simulink model "Robot4"  (R2018a)
settings: Solver=VariableStepAuto  StartTime=0.0  StopTime=10.0  RelTol=1e-3
settings Model: Creator=Carapinha  LastModifiedBy=Carapinha

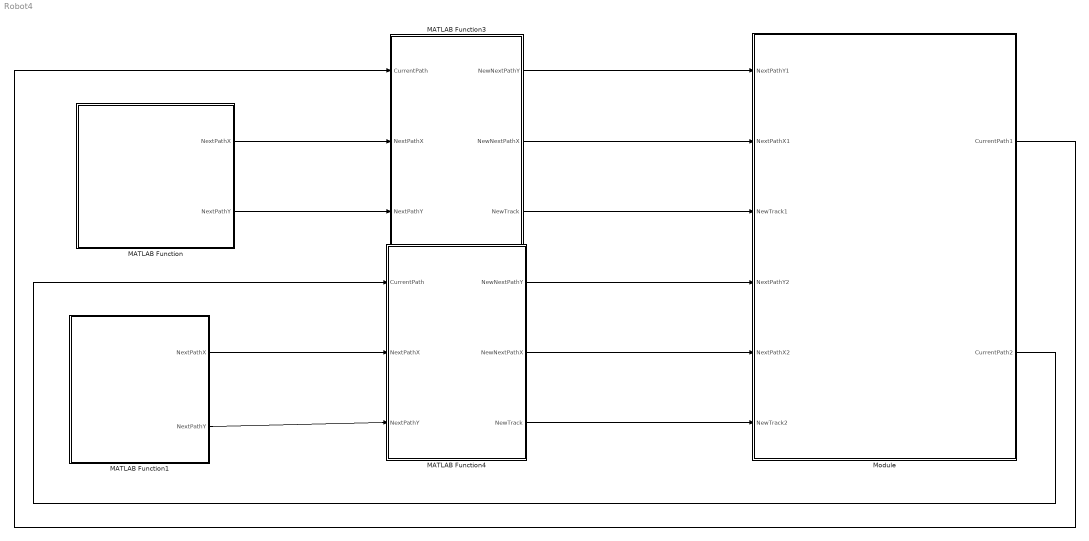
== system Robot4 ==
  MATLAB Function : MATLAB Function  TreatAsAtomicUnit=on
  MATLAB Function1 : MATLAB Function  TreatAsAtomicUnit=on
  MATLAB Function3 : MATLAB Function  TreatAsAtomicUnit=on
  MATLAB Function4 : MATLAB Function  TreatAsAtomicUnit=on
  Module : Stateflow chart  TreatAsAtomicUnit=on
  wires:
  MATLAB Function4/2(NewNextPathX) -> Module/5(NextPathX2)
  MATLAB Function4/1(NewNextPathY) -> Module/4(NextPathY2)
  MATLAB Function3/3(NewTrack) -> Module/3(NewTrack1)
  MATLAB Function1/2(NextPathY) -> MATLAB Function4/3(NextPathY)
  MATLAB Function3/1(NewNextPathY) -> Module/1(NextPathY1)
  MATLAB Function3/2(NewNextPathX) -> Module/2(NextPathX1)
  MATLAB Function1/1(NextPathX) -> MATLAB Function4/2(NextPathX)
  MATLAB Function/2(NextPathY) -> MATLAB Function3/3(NextPathY)
  Module/1(CurrentPath1) -> MATLAB Function3/1(CurrentPath)
  Module/2(CurrentPath2) -> MATLAB Function4/1(CurrentPath)
  MATLAB Function/1(NextPathX) -> MATLAB Function3/2(NextPathX)
  MATLAB Function4/3(NewTrack) -> Module/6(NewTrack2)

== matlab function Robot4/MATLAB Function1 ==
  data: NextPathX output; NextPathY output
function [NextPathX, NextPathY] = RandomPath()
    NextPathX = round(rand(1)*2-1);
    NextPathY = round(rand(1)*2-1);
    return
end

== matlab function Robot4/MATLAB Function ==
  data: NextPathX output; NextPathY output
function [NextPathX, NextPathY] = RandomPath()
    NextPathX = round(rand(1)*2-1);
    NextPathY = round(rand(1)*2-1);
    return
end

== stateflow chart Robot4/Module ==
  state Main
    state Robot1 [parallel]
      settings: executionOrder=1
      state StopR1
        entry:
        %PathBlocked
        Move1 = 1;
        Stop1 = 0;
      state MoveR1
        entry:
        Car1 = 1;
        Move1 = 0;
        Stop1 = 1;
      StopR1 -> MoveR1 [order 1] : [NewTrack1 == CurrentTrack2]
      (default) -> MoveR1
      MoveR1 -> StopR1 : [NewTrack1 ~= CurrentTrack2]
      StopR1 -> StopR1 [order 2] : [after(1,sec)]
    state Controller1 [parallel]
      settings: executionOrder=2
      state E
        entry:
        A(5,1) = 1;
        CurrentPath1 = 5;
        exit:
        A(5,1) = 0;
      state I
        entry:
        A(4,2) = 1;
        CurrentPath1 = 9;
        exit:
        A(4,2) = 0;
      state O
        entry:
        A(5,3) = 1;
        CurrentPath1 = 15;
        exit:
        A(5,3) = 0;
      state C
        entry:
        A(3,1) = 1;
        CurrentPath1 = 3;
        exit:
        A(3,1) = 0;
      state Start1
        entry:
      state S
        entry:
        A(4,4) = 1;
        CurrentPath1 = 19;
        exit:
        A(4,4) = 0;
      state A
        entry:
        A(1,1) = 1;
        CurrentPath1 = 1;
        exit:
        A(1,1) = 0;
      state G
        entry:
        A(2,2) = 1;
        CurrentPath1 = 7;
        exit:
        A(2,2) = 0;
      state M
        entry:
        A(3,3) = 1;
        CurrentPath1 = 13;
        exit:
        A(3,3) = 0;
      state Z
        entry:
        A(5,5) = 1;
        CurrentPath1 = 25;
        exit:
        A(5,5) = 0;
      state K
        entry:
        A(1,3) = 1;
        CurrentPath1 = 11;
        exit:
        A(1,3) = 0;
      state Q
        entry:
        A(2,4) = 1;
        CurrentPath1 = 17;
        exit:
        A(2,4) = 0;
      state X
        entry:
        A(3,5) = 1;
        CurrentPath1 = 23;
        exit:
        A(3,5) = 0;
      state U
        entry:
        A(1,5) = 1;
        CurrentPath1 = 21;
        exit:
        A(1,5) = 0;
      E -> Main.Controller1.I : [Move1 == 1 && NextPathX1 == -1 && NextPathY1 == -1]
      Main.Controller1.I -> E [order 2] : [Move1 == 1 && NextPathX1 == 1 && NextPathY1 == 1]
      (default) -> Start1
      Main.Controller1.C -> Main.Controller1.I [order 2] : [Move1 == 1 && NextPathX1 == 1 && NextPathY1 == -1]
      Main.Controller1.I -> Main.Controller1.O [order 3] : [Move1 == 1 && NextPathX1 == 1 && NextPathY1 == -1]
      Main.Controller1.I -> Main.Controller1.C [order 1] : [Move1 == 1 && NextPathX1 == -1 && NextPathY1 == 1]
      Main.Controller1.O -> Main.Controller1.I [order 1] : [Move1 == 1 && NextPathX1 == -1 && NextPathY1 == 1]
      Main.Controller1.C -> Main.Controller1.G [order 1] : [Move1 == 1 && NextPathX1 == -1 && NextPathY1 == -1]
      Main.Controller1.G -> Main.Controller1.C [order 2] : [Move1 == 1 && NextPathX1 == 1 && NextPathY1 == 1]
      Main.Controller1.O -> Main.Controller1.S [order 2] : [Move1 == 1 && NextPathX1 == -1 && NextPathY1 == -1]
      Main.Controller1.S -> Main.Controller1.O [order 2] : [Move1 == 1 && NextPathX1 == 1 && NextPathY1 == 1]
      Main.Controller1.I -> Main.Controller1.M [order 4] : [Move1 == 1 && NextPathX1 == -1 && NextPathY1 == -1]
      Main.Controller1.M -> Main.Controller1.I [order 1] : [Move1 == 1 && NextPathX1 == 1 && NextPathY1 == 1]
      Start1 -> Main.Controller1.A : [Car1 == 1]
      Main.Controller1.G -> Main.Controller1.M [order 3] : [Move1 == 1 && NextPathX1 == 1 && NextPathY1 == -1]
      Main.Controller1.A -> Main.Controller1.G : [Move1 == 1 && NextPathX1 == 1 && NextPathY1 == -1]
      Main.Controller1.S -> Main.Controller1.Z [order 3] : [Move1 == 1 && NextPathX1 == -1 && NextPathY1 == -1]
      Main.Controller1.S -> Main.Controller1.M [order 4] : [Move1 == 1 && NextPathX1 == -1 && NextPathY1 == 1]
      Main.Controller1.G -> Main.Controller1.A [order 1] : [Move1 == 1 && NextPathX1 == -1 && NextPathY1 == 1]
      Main.Controller1.M -> Main.Controller1.G [order 4] : [Move1 == 1 && NextPathX1 == -1 && NextPathY1 == 1]
      Main.Controller1.Z -> Main.Controller1.S : [Move1 == 1 && NextPathX1 == -1 && NextPathY1 == 1]
      Main.Controller1.M -> Main.Controller1.S [order 2] : [Move1 == 1 && NextPathX1 == 1 && NextPathY1 == -1]
      Main.Controller1.G -> Main.Controller1.K [order 4] : [Move1 == 1 && NextPathX1 == -1 && NextPathY1 == -1]
      Main.Controller1.K -> Main.Controller1.G [order 1] : [Move1 == 1 && NextPathX1 == 1 && NextPathY1 == 1]
      Main.Controller1.S -> Main.Controller1.X [order 1] : [Move1 == 1 && NextPathX1 == -1 && NextPathY1 == -1]
      Main.Controller1.X -> Main.Controller1.S [order 2] : [Move1 == 1 && NextPathX1 == 1 && NextPathY1 == 1]
      Main.Controller1.M -> Main.Controller1.Q [order 3] : [Move1 == 1 && NextPathX1 == -1 && NextPathY1 == -1]
      Main.Controller1.Q -> Main.Controller1.M [order 1] : [Move1 == 1 && NextPathX1 == 1 && NextPathY1 == 1]
      Main.Controller1.K -> Main.Controller1.Q [order 2] : [Move1 == 1 && NextPathX1 == 1 && NextPathY1 == -1]
      Main.Controller1.X -> Main.Controller1.Q [order 1] : [Move1 == 1 && NextPathX1 == -1 && NextPathY1 == 1]
      Main.Controller1.Q -> Main.Controller1.K [order 3] : [Move1 == 1 && NextPathX1 == -1 && NextPathY1 == 1]
      Main.Controller1.Q -> Main.Controller1.X [order 2] : [Move1 == 1 && NextPathX1 == 1 && NextPathY1 == -1]
      Main.Controller1.Q -> Main.Controller1.U [order 4] : [Move1 == 1 && NextPathX1 == -1 && NextPathY1 == -1]
      Main.Controller1.U -> Main.Controller1.Q : [Move1 == 1 && NextPathX1 == 1 && NextPathY1 == 1]
    state Robot4 [parallel]
      settings: executionOrder=3
      state StopR2
        entry:
        %PathBlocked
        Move2 = 1;
        Stop2 = 0;
      state MoveR2
        entry:
        Car2 = 1;
        Move2 = 0;
        Stop2 = 1;
      StopR2 -> MoveR2 [order 1] : [NewTrack2 == CurrentTrack1]
      (default) -> MoveR2
      MoveR2 -> StopR2 : [NewTrack2 ~= CurrentTrack1]
      StopR2 -> StopR2 [order 2] : [after(1,sec)]
    state Controller1 [parallel]
      settings: executionOrder=4
      state E1
        entry:
        A(5,1) = 2;
        CurrentPath2 = 5;
        exit:
        A(5,1) = 0;
      state C
        entry:
        A(3,1) = 2;
        CurrentPath2 = 3;
        exit:
        A(3,1) = 0;
      state I
        entry:
        A(4,2) = 2;
        CurrentPath2 = 9;
        exit:
        A(4,2) = 0;
      state O
        entry:
        A(5,3) = 2;
        CurrentPath2 = 15;
        exit:
        A(5,3) = 0;
      state Start2
        entry:
      state A
        entry:
        A(1,1) = 2;
        CurrentPath2 = 1;
        exit:
        A(1,1) = 0;
      state G
        entry:
        A(2,2) = 2;
        CurrentPath2 = 7;
        exit:
        A(2,2) = 0;
      state S
        entry:
        A(4,4) = 2;
        CurrentPath2 = 19;
        exit:
        A(4,4) = 0;
      state M
        entry:
        A(3,3) = 2;
        CurrentPath2 = 13;
        exit:
        A(3,3) = 0;
      state Z
        entry:
        A(5,5) = 2;
        CurrentPath2 = 25;
        exit:
        A(5,5) = 0;
      state Q
        entry:
        A(2,4) = 2;
        CurrentPath2 = 17;
        exit:
        A(2,4) = 0;
      state X
        entry:
        A(3,5) = 2;
        CurrentPath2 = 23;
        exit:
        A(3,5) = 0;
      state K
        entry:
        A(1,3) = 2;
        CurrentPath2 = 11;
        exit:
        A(1,3) = 0;
      state U
        entry:
        A(1,5) = 2;
        CurrentPath2 = 21;
        exit:
        A(1,5) = 0;
      Main.Controller1.I -> E1 [order 2] : [Move2 == 1 && NextPathX2 == 1 && NextPathY2 == 1]
      E1 -> Main.Controller1.I : [Move2 == 1 && NextPathX2 == -1 && NextPathY2 == -1]
      Main.Controller1.C -> Main.Controller1.I [order 2] : [Move2 == 1 && NextPathX2 == 1 && NextPathY2 == -1]
      (default) -> Start2
      Main.Controller1.I -> Main.Controller1.C [order 1] : [Move2 == 1 && NextPathX2 == -1 && NextPathY2 == 1]
      Main.Controller1.I -> Main.Controller1.O [order 3] : [Move2 == 1 && NextPathX2 == 1 && NextPathY2 == -1]
      Main.Controller1.C -> Main.Controller1.G [order 1] : [Move2 == 1 && NextPathX2 == -1 && NextPathY2 == -1]
      Main.Controller1.G -> Main.Controller1.C [order 2] : [Move2 == 1 && NextPathX2 == 1 && NextPathY2 == 1]
      Main.Controller1.O -> Main.Controller1.I [order 1] : [Move2 == 1 && NextPathX2 == -1 && NextPathY2 == 1]
      Main.Controller1.O -> Main.Controller1.S [order 2] : [Move2 == 1 && NextPathX2 == -1 && NextPathY2 == -1]
      Main.Controller1.S -> Main.Controller1.O [order 2] : [Move2 == 1 && NextPathX2 == 1 && NextPathY2 == 1]
      Main.Controller1.I -> Main.Controller1.M [order 4] : [Move2 == 1 && NextPathX2 == -1 && NextPathY2 == -1]
      Main.Controller1.M -> Main.Controller1.I [order 1] : [Move2 == 1 && NextPathX2 == 1 && NextPathY2 == 1]
      Start2 -> Main.Controller1.Z : [Car2 == 1]
      Main.Controller1.A -> Main.Controller1.G : [Move2 == 1 && NextPathX2 == 1 && NextPathY2 == -1]
      Main.Controller1.G -> Main.Controller1.M [order 3] : [Move2 == 1 && NextPathX2 == 1 && NextPathY2 == -1]
      Main.Controller1.G -> Main.Controller1.A [order 1] : [Move2 == 1 && NextPathX2 == -1 && NextPathY2 == 1]
      Main.Controller1.S -> Main.Controller1.M [order 4] : [Move2 == 1 && NextPathX2 == -1 && NextPathY2 == 1]
      Main.Controller1.S -> Main.Controller1.Z [order 3] : [Move2 == 1 && NextPathX2 == -1 && NextPathY2 == -1]
      Main.Controller1.M -> Main.Controller1.G [order 4] : [Move2 == 1 && NextPathX2 == -1 && NextPathY2 == 1]
      Main.Controller1.M -> Main.Controller1.S [order 2] : [Move2 == 1 && NextPathX2 == 1 && NextPathY2 == -1]
      Main.Controller1.Z -> Main.Controller1.S : [Move2 == 1 && NextPathX2 == -1 && NextPathY2 == 1]
      Main.Controller1.G -> Main.Controller1.K [order 4] : [Move2 == 1 && NextPathX2 == -1 && NextPathY2 == -1]
      Main.Controller1.K -> Main.Controller1.G [order 1] : [Move2 == 1 && NextPathX2 == 1 && NextPathY2 == 1]
      Main.Controller1.M -> Main.Controller1.Q [order 3] : [Move2 == 1 && NextPathX2 == -1 && NextPathY2 == -1]
      Main.Controller1.Q -> Main.Controller1.M [order 1] : [Move2 == 1 && NextPathX2 == 1 && NextPathY2 == 1]
      Main.Controller1.S -> Main.Controller1.X [order 1] : [Move2 == 1 && NextPathX2 == -1 && NextPathY2 == -1]
      Main.Controller1.X -> Main.Controller1.S [order 2] : [Move2 == 1 && NextPathX2 == 1 && NextPathY2 == 1]
      Main.Controller1.Q -> Main.Controller1.K [order 3] : [Move2 == 1 && NextPathX2 == -1 && NextPathY2 == 1]
      Main.Controller1.X -> Main.Controller1.Q [order 1] : [Move2 == 1 && NextPathX2 == -1 && NextPathY2 == 1]
      Main.Controller1.Q -> Main.Controller1.X [order 2] : [Move2 == 1 && NextPathX2 == 1 && NextPathY2 == -1]
      Main.Controller1.K -> Main.Controller1.Q [order 2] : [Move2 == 1 && NextPathX2 == 1 && NextPathY2 == -1]
      Main.Controller1.Q -> Main.Controller1.U [order 4] : [Move2 == 1 && NextPathX2 == -1 && NextPathY2 == -1]
      Main.Controller1.U -> Main.Controller1.Q : [Move2 == 1 && NextPathX2 == 1 && NextPathY2 == 1]
  (default) -> Main
  data: Permission2 local =0; Decel local; Accel local; NextPathY1 input =0; NextPathX1 input; NewTrack1 input; NextPathY2 input =0; close3 local; Enter3 local; LeftC3 local; Stop3 local; Permission3 local =0; LeftC local; close local; cp local; LeftC2 local; cp2 local; Enter local; Stop local; close2 local; Stop2 local; Enter2 local; cp3 local; NextPathX2 input =0; NewTrack2 input; CurrentPath1 output; CurrentPath2 output

== matlab function Robot4/MATLAB Function3 ==
  data: CurrentPath input; NewNextPathY output; NextPathX input; NextPathY input; NewNextPathX output; NewTrack output
function [NewNextPathY, NewNextPathX, NewTrack] = CheckPath(CurrentPath, NextPathX, NextPathY)

NewNextPathY = NextPathY;
NewNextPathX = NextPathX;
%Fix invalid Y NextPath
if(CurrentPath == 1 || CurrentPath == 3 || CurrentPath == 5)
    if(NextPathY == 1)
        NewNextPathY = -1;
        NewNextPathX = NextPathX;
    end
end

if(CurrentPath == 21 || CurrentPath == 23 ||CurrentPath == 25)
    if(NextPathY == -1)
        NewNextPathY = 1;
        NewNextPathX = NextPathX;
    end
end

%Fix invalid X NextPath
if(CurrentPath == 1 || CurrentPath == 11 || CurrentPath == 21)
    if(NextPathX == -1)
        NewNextPathX = 1;
        NewNextPathY = NextPathY;
    end
end

if(CurrentPath == 5 || CurrentPath == 15 || CurrentPath == 25)
    if(NextPathX == 1)
        NewNextPathX = -1;
        NewNextPathY = NextPathY;
    end
end

switch CurrentPath
    case 1 %A
        if (NewNextPathY == -1 && NewNextPathX == 1)
            NewTrack = 7;
        end
    case 3 %C
        if (NewNextPathY == -1 && NewNextPathX == 1)
            NewTrack = 9;
        elseif (NewNextPathY == -1 && NewNextPathX == -1)
            NewTrack = 7;
        end
    case 5 %E
        if (NewNextPathY == -1 && NewNextPathX == -1)
            NewTrack = 9;
        end
    case 7 %G
        if (NewNextPathY == -1 && NewNextPathX == -1)
            NewTrack = 11;
        elseif (NewNextPathY == 1 && NewNextPathX == 1)
            NewTrack = 3;
        elseif (NewNextPathY == -1 && NewNextPathX == 1)
            NewTrack = 13;
        elseif (NewNextPathY == 1 && NewNextPathX == -1)
            NewTrack = 1;
        end
    case 9 %I
        if (NewNextPathY == -1 && NewNextPathX == -1)
            NewTrack = 13;
        elseif (NewNextPathY == 1 && NewNextPathX == 1)
            NewTrack = 5;
        elseif (NewNextPathY == -1 && NewNextPathX == 1)
            NewTrack = 15;
        elseif (NewNextPathY == 1 && NewNextPathX == -1)
            NewTrack = 3;
        end
    case 11 %K
        if (NewNextPathY == -1 && NewNextPathX == 1)
            NewTrack = 17;
        elseif (NewNextPathY == 1 && NewNextPathX == 1)
            NewTrack = 7;
        end
    case 13 %M
        if (NewNextPathY == -1 && NewNextPathX == -1)
            NewTrack = 17;
        elseif (NewNextPathY == 1 && NewNextPathX == 1)
            NewTrack = 9;
        elseif (NewNextPathY == -1 && NewNextPathX == 1)
            NewTrack = 19;
        elseif (NewNextPathY == 1 && NewNextPathX == -1)
            NewTrack = 7;
        end
    case 15 %O
        if (NewNextPathY == 1 && NewNextPathX == -1)
            NewTrack = 9;
        elseif (NewNextPathY == -1 && NewNextPathX == -1)
            NewTrack = 19;
        end
    case 17 %Q
        if (NewNextPathY == -1 && NewNextPathX == -1)
            NewTrack = 21;
        elseif (NewNextPathY == 1 && NewNextPathX == 1)
            NewTrack = 13;
        elseif (NewNextPathY == -1 && NewNextPathX == 1)
            NewTrack = 23;
        elseif (NewNextPathY == 1 && NewNextPathX == -1)
            NewTrack = 11;
        end
    case 19 %S
        if (NewNextPathY == -1 && NewNextPathX == -1)
            NewTrack = 23;
        elseif (NewNextPathY == 1 && NewNextPathX == 1)
            NewTrack = 15;
        elseif (NewNextPathY == -1 && NewNextPathX == 1)
            NewTrack = 25;
        elseif (NewNextPathY == 1 && NewNextPathX == -1)
            NewTrack = 13;
        end
    case 21 %U
        if (NewNextPathY == 1 && NewNextPathX == 1)
            NewTrack = 17;
        end
    case 23 %X
        if (NewNextPathY == 1 && NewNextPathX == 1)
            NewTrack = 19;
        elseif (NewNextPathY == 1 && NewNextPathX == -1)
            NewTrack = 17;
        end
    case 25 %Z
        if (NewNextPathY == 1 && NewNextPathX == -1)
            NewTrack = 19;
        end
end
end

== matlab function Robot4/MATLAB Function4 ==
  data: CurrentPath input; NewNextPathY output; NextPathX input; NextPathY input; NewNextPathX output; NewTrack output
function [NewNextPathY, NewNextPathX, NewTrack] = CheckPath(CurrentPath, NextPathX, NextPathY)

NewNextPathY = NextPathY;
NewNextPathX = NextPathX;
%Fix invalid Y NextPath
if(CurrentPath == 1 || CurrentPath == 3 || CurrentPath == 5)
    if(NextPathY == 1)
        NewNextPathY = -1;
        NewNextPathX = NextPathX;
    end
end

if(CurrentPath == 21 || CurrentPath == 23 ||CurrentPath == 25)
    if(NextPathY == -1)
        NewNextPathY = 1;
        NewNextPathX = NextPathX;
    end
end

%Fix invalid X NextPath
if(CurrentPath == 1 || CurrentPath == 11 || CurrentPath == 21)
    if(NextPathX == -1)
        NewNextPathX = 1;
        NewNextPathY = NextPathY;
    end
end

if(CurrentPath == 5 || CurrentPath == 15 || CurrentPath == 25)
    if(NextPathX == 1)
        NewNextPathX = -1;
        NewNextPathY = NextPathY;
    end
end

switch CurrentPath
    case 1 %A
        if (NewNextPathY == -1 && NewNextPathX == 1)
            NewTrack = 7;
        end
    case 3 %C
        if (NewNextPathY == -1 && NewNextPathX == 1)
            NewTrack = 9;
        elseif (NewNextPathY == -1 && NewNextPathX == -1)
            NewTrack = 7;
        end
    case 5 %E
        if (NewNextPathY == -1 && NewNextPathX == -1)
            NewTrack = 9;
        end
    case 7 %G
        if (NewNextPathY == -1 && NewNextPathX == -1)
            NewTrack = 11;
        elseif (NewNextPathY == 1 && NewNextPathX == 1)
            NewTrack = 3;
        elseif (NewNextPathY == -1 && NewNextPathX == 1)
            NewTrack = 13;
        elseif (NewNextPathY == 1 && NewNextPathX == -1)
            NewTrack = 1;
        end
    case 9 %I
        if (NewNextPathY == -1 && NewNextPathX == -1)
            NewTrack = 13;
        elseif (NewNextPathY == 1 && NewNextPathX == 1)
            NewTrack = 5;
        elseif (NewNextPathY == -1 && NewNextPathX == 1)
            NewTrack = 15;
        elseif (NewNextPathY == 1 && NewNextPathX == -1)
            NewTrack = 3;
        end
    case 11 %K
        if (NewNextPathY == -1 && NewNextPathX == 1)
            NewTrack = 17;
        elseif (NewNextPathY == 1 && NewNextPathX == 1)
            NewTrack = 7;
        end
    case 13 %M
        if (NewNextPathY == -1 && NewNextPathX == -1)
            NewTrack = 17;
        elseif (NewNextPathY == 1 && NewNextPathX == 1)
            NewTrack = 9;
        elseif (NewNextPathY == -1 && NewNextPathX == 1)
            NewTrack = 19;
        elseif (NewNextPathY == 1 && NewNextPathX == -1)
            NewTrack = 7;
        end
    case 15 %O
        if (NewNextPathY == 1 && NewNextPathX == -1)
            NewTrack = 9;
        elseif (NewNextPathY == -1 && NewNextPathX == -1)
            NewTrack = 19;
        end
    case 17 %Q
        if (NewNextPathY == -1 && NewNextPathX == -1)
            NewTrack = 21;
        elseif (NewNextPathY == 1 && NewNextPathX == 1)
            NewTrack = 13;
        elseif (NewNextPathY == -1 && NewNextPathX == 1)
            NewTrack = 23;
        elseif (NewNextPathY == 1 && NewNextPathX == -1)
            NewTrack = 11;
        end
    case 19 %S
        if (NewNextPathY == -1 && NewNextPathX == -1)
            NewTrack = 23;
        elseif (NewNextPathY == 1 && NewNextPathX == 1)
            NewTrack = 15;
        elseif (NewNextPathY == -1 && NewNextPathX == 1)
            NewTrack = 25;
        elseif (NewNextPathY == 1 && NewNextPathX == -1)
            NewTrack = 13;
        end
    case 21 %U
        if (NewNextPathY == 1 && NewNextPathX == 1)
            NewTrack = 17;
        end
    case 23 %X
        if (NewNextPathY == 1 && NewNextPathX == 1)
            NewTrack = 19;
        elseif (NewNextPathY == 1 && NewNextPathX == -1)
            NewTrack = 17;
        end
    case 25 %Z
        if (NewNextPathY == 1 && NewNextPathX == -1)
            NewTrack = 19;
        end
end
end
